simulink model "Continuous_Time_STR"  (R2023a)
settings: Solver=FixedStepAuto  StartTime=start_time  StopTime=stop_time  FixedStep=sample_time  RelTol=1e-3
values from neighbouring files (symbols this model uses):
  a = H.Denominator{1}    [example4.m]    (also in example6.m = 1)
  b = H.Numerator{1}    [example4.m]    (also in example6.m = 1)
  W = 1    [example6.m]
  Z = 0.7    [example6.m]
settings Model: Creator=Mmoha  LastModifiedBy=Mmoha

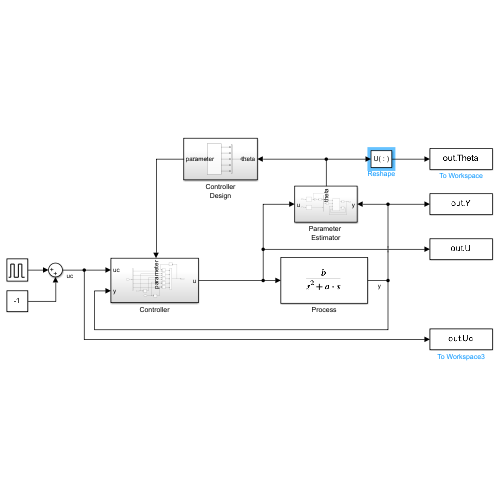
[thumbnail: Simulink's stored preview of the top-level diagram]
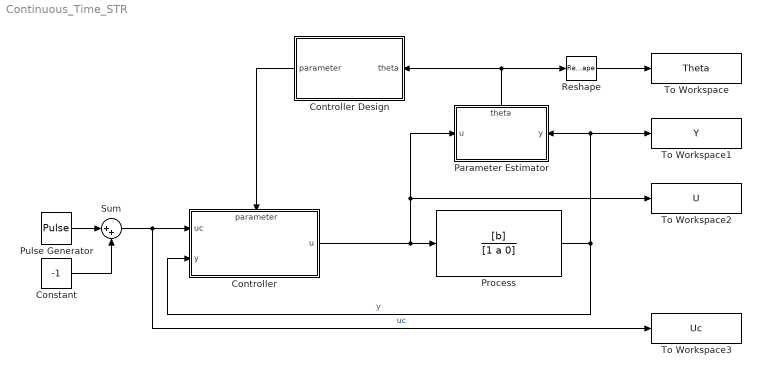
== system Continuous_Time_STR ==
  Constant : Constant  Value=-1
  Controller : Subsystem
      settings: PortSchema="{\"entries\":[{\"content\":{\"sides\":[{\"content\":{\"connectorIds\":[\"In1\",\"In2\"]},\"type\":\"ConnectorPlacement.EquallySpacedRectSide\",\"uuid\":\"c7578673-2701-46d0-8f3b-643132126a27\"},{\"content\":{\"connectorIds\":[\"Out1\"],\"side\":\"RIGHT\"},\"type\":\"ConnectorPlacement.EquallySpacedRectSide\",\"uuid\":\"d983a872-f9db-4cb9-8484-10da0d2a1e0a\"},{\"content\":{\"connectorIds\":[\"In3\"],\"side\":\"TOP\"},\"type\":\"ConnectorPlacement.EquallySpacedRectSide\",\"uuid\":\"af821799-924d-4122-a0c1-87cc58198574\"}]},\"type\":\"ConnectorPlacement.EquallySpacedConnector\",\"uuid\":\"ec2b55ff-1c53-425c-a5d2-aef2ec9dd43c\"}],\"packageUris\":[\"http://schema.mathworks.com/mf0/Connector/R2020b\"],\"version\":\"1.0\"}"
  Controller Design : Subsystem
      settings: PortSchema="{\"entries\":[{\"content\":{\"sides\":[{\"content\":{\"connectorIds\":[\"Out1\"]},\"type\":\"ConnectorPlacement.EquallySpacedRectSide\",\"uuid\":\"58baf7c7-d8e5-457e-9a16-6ffd3cafe73e\"},{\"content\":{\"connectorIds\":[\"In1\"],\"side\":\"RIGHT\"},\"type\":\"ConnectorPlacement.EquallySpacedRectSide\",\"uuid\":\"4da50bc7-c28e-4e6a-a02c-3014d7cddf80\"},{\"content\":{\"side\":\"TOP\"},\"type\":\"ConnectorPlacement.EquallySpacedRectSide\",\"uuid\":\"1ef2d438-976b-452b-977a-91e341f8ee1b\"},{\"content\":{\"side\":\"BOTTOM\"},\"type\":\"ConnectorPlacement.EquallySpacedRectSide\",\"uuid\":\"52580118-6ca9-4510-b3f9-d2a2c87850da\"}]},\"type\":\"ConnectorPlacement.EquallySpacedConnector\",\"uuid\":\"da256936-6820-4087-8ea1-33167bc1ce16\"}],\"packageUris\":[\"http://schema.mathworks.com/mf0/Connector/R2020b\"],\"version\":\"1.0\"}"
  Parameter Estimator : Subsystem
      settings: PortSchema="{\"entries\":[{\"content\":{\"sides\":[{\"content\":{\"connectorIds\":[\"In1\"]},\"type\":\"ConnectorPlacement.EquallySpacedRectSide\",\"uuid\":\"bbd79f27-b198-4510-be87-e6491af917de\"},{\"content\":{\"connectorIds\":[\"In2\"],\"side\":\"RIGHT\"},\"type\":\"ConnectorPlacement.EquallySpacedRectSide\",\"uuid\":\"b3ff166f-b811-4ca0-a53c-c9677dfa5441\"},{\"content\":{\"connectorIds\":[\"Out1\"],\"side\":\"TOP\"},\"type\":\"ConnectorPlacement.EquallySpacedRectSide\",\"uuid\":\"16147e99-6393-471b-8b17-a17587dcba86\"}]},\"type\":\"ConnectorPlacement.EquallySpacedConnector\",\"uuid\":\"adf548bb-ec4f-48e2-9ef8-4e2e411756c5\"}],\"packageUris\":[\"http://schema.mathworks.com/mf0/Connector/R2020b\"],\"version\":\"1.0\"}"
  Process : TransferFcn  Numerator=[b]  Denominator=[1 a 0]
  Pulse Generator : DiscretePulseGenerator  PulseType=Time based  Amplitude=2  Period=50  PulseWidth=50
  Reshape : Reshape
  Sum : Sum  Inputs=|++
  To Workspace : ToWorkspace  VariableName=Theta  SaveFormat=Timeseries  SampleTime=-1
  To Workspace1 : ToWorkspace  VariableName=Y  SaveFormat=Timeseries  SampleTime=-1
  To Workspace2 : ToWorkspace  VariableName=U  SaveFormat=Timeseries  SampleTime=-1
  To Workspace3 : ToWorkspace  VariableName=Uc  SaveFormat=Timeseries  SampleTime=-1
  wires:
  Pulse Generator/1 -> Sum/1
  Constant/1 -> Sum/2
  Process/1 -> To Workspace1/1, Parameter Estimator/2(y), Controller/2(y)  "y"
  Controller/1(u) -> Parameter Estimator/1(u), To Workspace2/1, Process/1
  Sum/1 -> To Workspace3/1, Controller/1(uc)  "uc"
  Parameter Estimator/1(theta) -> Controller Design/1(theta), Reshape/1
  Controller Design/1(parameter) -> Controller/3(parameter)
  Reshape/1 -> To Workspace/1

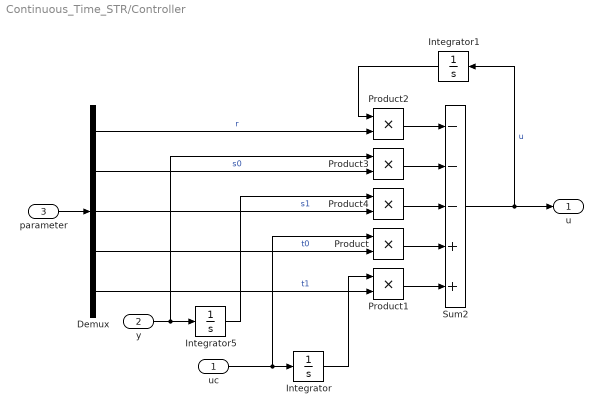
== system Continuous_Time_STR/Controller ==
  uc : Inport
  y : Inport  Port=2
  parameter : Inport  Port=3
  Demux : Demux  Outputs=5
  Integrator : Integrator
  Integrator1 : Integrator
  Integrator5 : Integrator
  Product{,1..4} (5 alike) : Product
  Sum2 : Sum  Inputs=---++
  u : Outport
  wires:
  uc/1 -> Integrator/1, Product/1
  y/1 -> Product3/1, Integrator5/1
  Sum2/1 -> Integrator1/1, u/1  "u"
  parameter/1 -> Demux/1
  Product1/1 -> Sum2/5
  Integrator5/1 -> Product4/1
  Demux/2 -> Product3/2  "s0"
  Demux/1 -> Product2/2  "r"
  Product4/1 -> Sum2/3
  Product3/1 -> Sum2/2
  Demux/5 -> Product1/2  "t1"
  Demux/4 -> Product/2  "t0"
  Integrator1/1 -> Product2/1
  Demux/3 -> Product4/2  "s1"
  Product2/1 -> Sum2/1
  Integrator/1 -> Product1/1
  Product/1 -> Sum2/4

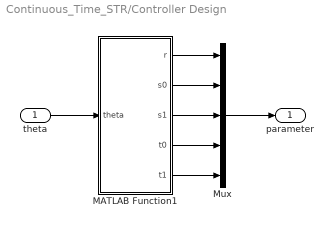
== system Continuous_Time_STR/Controller Design ==
  theta : Inport
  MATLAB Function1 : MATLAB Function  TreatAsAtomicUnit=on
  Mux : Mux  Inputs=5
  parameter : Outport
  wires:
  theta/1 -> MATLAB Function1/1(theta)
  MATLAB Function1/3(s1) -> Mux/3
  MATLAB Function1/5(t1) -> Mux/5
  MATLAB Function1/2(s0) -> Mux/2
  MATLAB Function1/1(r) -> Mux/1
  Mux/1 -> parameter/1
  MATLAB Function1/4(t0) -> Mux/4

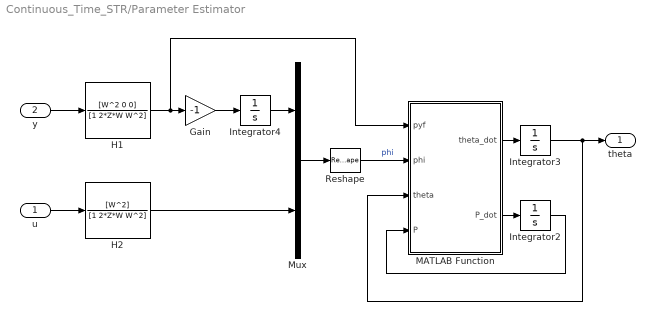
== system Continuous_Time_STR/Parameter Estimator ==
  u : Inport
  y : Inport  Port=2
  Gain : Gain  Gain=-1
  H1 : TransferFcn  Numerator=[W^2 0 0]  Denominator=[1 2*Z*W W^2]
  H2 : TransferFcn  Numerator=[W^2]  Denominator=[1 2*Z*W W^2]
  Integrator2 : Integrator  InitialCondition=100*eye(2)
  Integrator3 : Integrator  InitialCondition=[2 0.2]
  Integrator4 : Integrator
  MATLAB Function : MATLAB Function  TreatAsAtomicUnit=on
  Mux : Mux  Inputs=2
  Reshape : Reshape  OutputDimensionality=Column vector (2-D)
  theta : Outport
  wires:
  Integrator3/1 -> theta/1, MATLAB Function/3(theta)
  Integrator2/1 -> MATLAB Function/4(P)
  Integrator4/1 -> Mux/1
  MATLAB Function/2(P_dot) -> Integrator2/1
  H1/1 -> MATLAB Function/1(pyf), Gain/1
  H2/1 -> Mux/2
  Mux/1 -> Reshape/1
  MATLAB Function/1(theta_dot) -> Integrator3/1
  Gain/1 -> Integrator4/1
  Reshape/1 -> MATLAB Function/2(phi)  "phi"
  y/1 -> H1/1
  u/1 -> H2/1

== matlab function Continuous_Time_STR/Controller Design/MATLAB Function1 ==
  data: theta input; r output; s0 output; s1 output; t0 output; t1 output
function [r, s0 ,s1, t0, t1] = fcn(theta)
a = theta(1);
b = theta(2);
W = 1;
Z = 0.7;
a0 = 2;

Phi = [1 0 0; a b 0; 0 0 b];
Y = [2*Z*W+a0-a; 2*Z*W*a0+W^2; a0*W^2];
X = Phi\Y;
r = X(1);
s0 = X(2); 
s1 = X(3);
beta = W^2 / b;
t0 = beta;
t1 = beta*a0;

== matlab function Continuous_Time_STR/Parameter Estimator/MATLAB Function ==
  data: pyf input; theta_dot output; phi input; theta input; P input; P_dot output
function [theta_dot, P_dot] = fcn(pyf, phi, theta, P)
alpha = 0;
e = pyf - phi'*theta;
theta_dot = P*phi*e;
P_dot = alpha*P - P*(phi*phi')*P;
